simulink model "stuSimulation_tm_2ask_new"  (R2021a)
settings: Solver=VariableStepAuto  StartTime=0.0  StopTime=3  RelTol=1e-3
undefined symbols (not defined in the file or in its folder): doppler
libraries: dspsrcs4 x3, commchan3 x2, dspfdesign x1
settings Model: Creator=dm  LastModifiedBy=timingyang
settings SolverCC: AlgebraicLoopSolver=TrustRegion

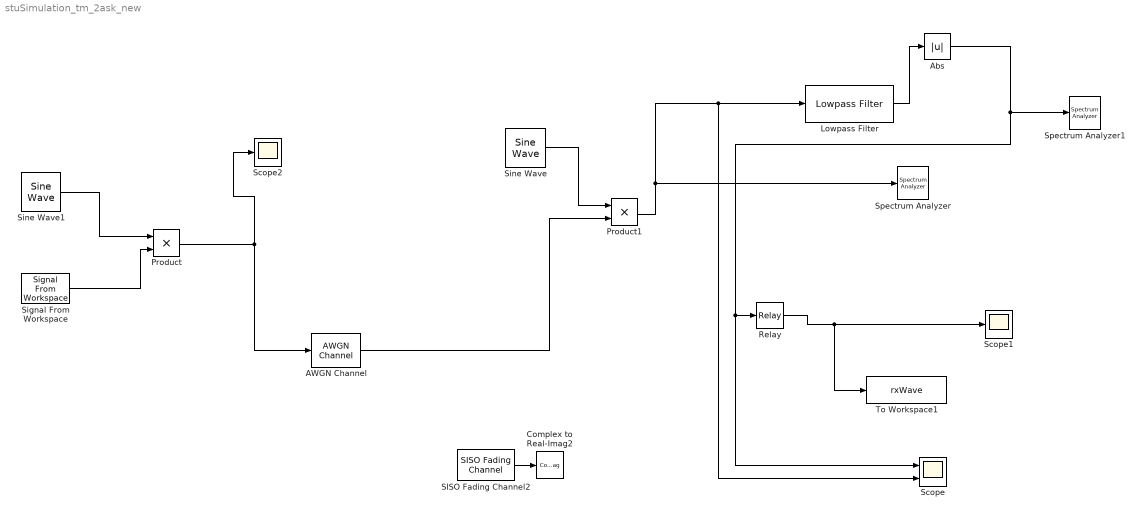
== system stuSimulation_tm_2ask_new ==
  AWGN Channel : commchan3/AWGN Channel  InputProcessing=Columns as channels (frame based)  seed=67  noiseMode="Signal to noise ratio  (Eb/No)"  EbNodB=25  EsNodB=10  SNRdB=10  bitsPerSym=1  Ps=1  Tsym=1e-3  variance=1
  Abs : Abs
  Complex to Real-Imag2 : ComplexToRealImag  Output=Real
  Lowpass Filter : dspfdesign/Lowpass Filter  FilterType=IIR  DesignForMinimumOrder=on  FilterOrder=50  PassbandFrequency=1000  StopbandFrequency=2000  PassbandRipple=0.1  StopbandAttenuation=60  InheritSampleRate=on  SampleRate=44100  SimulateUsing=Interpreted execution  roundingMode=Floor  coeffsDataTypeStr=fixdt(1,16)
  Product : Product  RndMeth=Zero
  Product1 : Product
  Relay : Relay  OnSwitchValue=0.25  OffSwitchValue=0.25
  SISO Fading Channel2 : commchan3/SISO Fading Channel  InheritSampleRate=on  SampleRate=1  PathDelays=0.001  AveragePathGains=-20  NormalizePathGains=on  FadingDistribution=Rician  KFactor=3  DirectPathDopplerShift=1  DirectPathInitialPhase=1  MaximumDopplerShift=2  DopplerSpectrum=doppler('Jakes')  RandomStream=mt19937ar with seed  Seed=73  PathGainsOutputPort=off  ChannelFilterDelayOutputPort=off  SimulateUsing=Interpreted execution  Visualization=Off  PathsForDopplerDisplay=1  SamplesToDisplay=25%
  Scope : Scope  NumInputPorts=2
  Scope1 : Scope
  Scope2 : Scope
  Signal From Workspace : dspsrcs4/Signal From Workspace  X=txWave  Ts=1/100e3  nsamps=20000  OutputAfterFinalValue=Cyclic repetition  ignoreOrWarnInputAndFrameLengths=on  OutputFrames=off
  Sine Wave : dspsrcs4/Sine Wave  Amplitude=1  Frequency=10000  Phase=0  SampleMode=Discrete  OutComplex=Real  CompMethod=Trigonometric fcn  TableSize=Speed  SampleTime=1/100e3  SamplesPerFrame=20000  ResetState=Restart at time zero  OutputFrames=off  dataType=double  wordLen=16  udDataType=sfix(16)  fracBitsMode=Best precision  numFracBits=15  OutDataTypeStr=double  LastOutDataTypeStr=double
  Sine Wave1 : dspsrcs4/Sine Wave  Amplitude=1  Frequency=10000  Phase=0  SampleMode=Discrete  OutComplex=Real  CompMethod=Table lookup  TableSize=Speed  SampleTime=1/100e3  SamplesPerFrame=20000  ResetState=Restart at time zero  OutputFrames=off  dataType=double  wordLen=16  udDataType=sfix(16)  fracBitsMode=Best precision  numFracBits=15  OutDataTypeStr=double  LastOutDataTypeStr=double
  Spectrum Analyzer : SpectrumAnalyzer
  Spectrum Analyzer1 : SpectrumAnalyzer
  To Workspace1 : ToWorkspace  VariableName=rxWave  SampleTime=1e-5
      settings: MaxDataPoints=1e5  Decimation=1e4
  wires:
  Relay/1 -> To Workspace1/1, Scope1/1
  Sine Wave/1 -> Product1/1
  Signal From Workspace/1 -> Product/2
  Sine Wave1/1 -> Product/1
  Product/1 -> AWGN Channel/1, Scope2/1
  Product1/1 -> Scope/2, Lowpass Filter/1, Spectrum Analyzer/1
  AWGN Channel/1 -> Product1/2
  Lowpass Filter/1 -> Abs/1
  Abs/1 -> Scope/1, Relay/1, Spectrum Analyzer1/1
  SISO Fading Channel2/1 -> Complex to Real-Imag2/1
